simulink model "q1_model2"  (R2018a)
settings: Solver=FixedStepAuto  StartTime=0.0  StopTime=t_f  FixedStep=1  RelTol=1e-3
values from neighbouring files (symbols this model uses):
  A = [100  0  0  -57.735026919; 0  100  0  -57.735026919; 0  0  100  -57.735026919]    [data.mat]    (also in q1.m = [h1_hat h2_hat h3_hat h4_hat])
  I_b = [100 1 2; 1 150 3; 2 3 200]    [q1.m]    (also in q3.m)
  Kd = -4    [q1.m]
  Kp = -.01    (= -0.01)    [q1.m]
  omega_B_N_t0 = zeros(3,1)    [q1.m]
  pinvA = pinv(A)    [q1.m]
  q_f = [q_f(2:4) q_f(1)].'    [q1.m]
  q_t0 = [0 0 0 1].'    [q1.m]    (also in q3.m)
libraries: vrlib x1
settings Model: Creator=Padraig Lysandrou  LastModifiedBy=Padraig Lysandrou

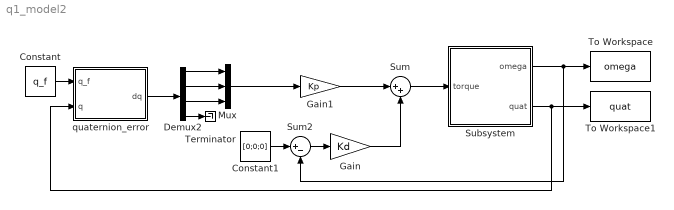
== system q1_model2 ==
  Constant : Constant  Value=q_f  VectorParams1D=off
  Constant1 : Constant  Value=[0;0;0]
  Demux2 : Demux
  Gain : Gain  Gain=Kd
  Gain1 : Gain  Gain=Kp
  Mux : Mux  Inputs=3
  Subsystem : Subsystem
  Sum : Sum  Inputs=|++
  Sum2 : Sum  Inputs=|+-
  Terminator : Terminator
  To Workspace : ToWorkspace  VariableName=omega  SaveFormat=Timeseries  SampleTime=-1
  To Workspace1 : ToWorkspace  VariableName=quat  SaveFormat=Timeseries  SampleTime=-1
  quaternion_error : MATLAB Function  TreatAsAtomicUnit=on
  wires:
  Sum/1 -> Subsystem/1(torque)
  Subsystem/1("omega ") -> Sum2/2, To Workspace/1
  Gain1/1 -> Sum/1
  Gain/1 -> Sum/2
  Constant1/1 -> Sum2/1
  Sum2/1 -> Gain/1
  Subsystem/2(quat) -> quaternion_error/2(q), To Workspace1/1
  Constant/1 -> quaternion_error/1(q_f)
  Demux2/3 -> Mux/3
  Demux2/1 -> Mux/1
  Demux2/4 -> Terminator/1
  Demux2/2 -> Mux/2
  quaternion_error/1(dq) -> Demux2/1
  Mux/1 -> Gain1/1

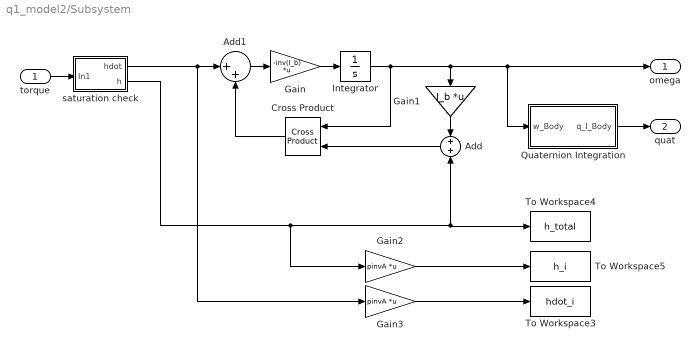
== system q1_model2/Subsystem ==
  torque : Inport
  Add : Sum
  Add1 : Sum  Inputs=|++
  Cross Product : vrlib/Utilities/Cross Product
      settings: SourceProductBaseCode=VR
  Gain : Gain  Gain=-inv(I_b)  Multiplication=Matrix(K*u) (u vector)
  Gain1 : Gain  Gain=I_b  Multiplication=Matrix(K*u) (u vector)
  Gain2 : Gain  Gain=pinvA  Multiplication=Matrix(K*u) (u vector)
  Gain3 : Gain  Gain=pinvA  Multiplication=Matrix(K*u) (u vector)
  Integrator : Integrator  InitialCondition=omega_B_N_t0
  Quaternion Integration : Subsystem
  To Workspace3 : ToWorkspace  VariableName=hdot_i  SaveFormat=Timeseries  SampleTime=-1
  To Workspace4 : ToWorkspace  VariableName=h_total  SaveFormat=Timeseries  SampleTime=-1
  To Workspace5 : ToWorkspace  VariableName=h_i  SaveFormat=Timeseries  SampleTime=-1
  saturation check : Subsystem
  "omega " : Outport
  quat : Outport  Port=2
  wires:
  Integrator/1 -> Quaternion Integration/1(w_Body), "omega "/1, Gain1/1, Cross Product/1
  Gain/1 -> Integrator/1
  Gain1/1 -> Add/1
  Add/1 -> Cross Product/2
  Add1/1 -> Gain/1
  Cross Product/1 -> Add1/2
  saturation check/2(h) -> Gain2/1, Add/2, To Workspace4/1
  Gain2/1 -> To Workspace5/1
  Gain3/1 -> To Workspace3/1
  Quaternion Integration/1(q_I_Body) -> quat/1
  torque/1 -> saturation check/1(In1)
  saturation check/1(hdot) -> Gain3/1, Add1/1

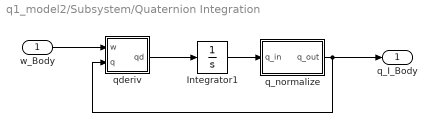
== system q1_model2/Subsystem/Quaternion Integration ==
  w_Body : Inport
  Integrator1 : Integrator  InitialCondition=q_t0
  q_normalize : Subsystem
  qderiv : Subsystem
  q_I_Body : Outport
  wires:
  w_Body/1 -> qderiv/1(w)
  q_normalize/1(q_out) -> qderiv/2(q), q_I_Body/1
  Integrator1/1 -> q_normalize/1(q_in)
  qderiv/1(qd) -> Integrator1/1

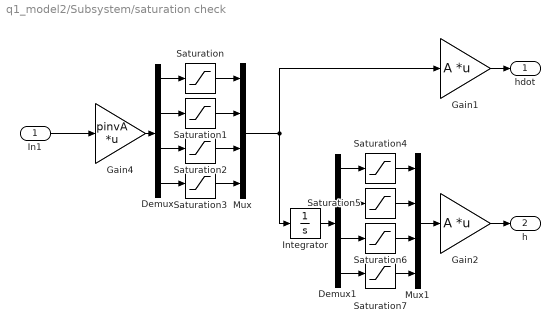
== system q1_model2/Subsystem/saturation check ==
  In1 : Inport
  Demux : Demux
  Demux1 : Demux
  Gain1 : Gain  Gain=A  Multiplication=Matrix(K*u) (u vector)
  Gain2 : Gain  Gain=A  Multiplication=Matrix(K*u) (u vector)
  Gain4 : Gain  Gain=pinvA  Multiplication=Matrix(K*u) (u vector)
  Integrator : Integrator
  Mux : Mux
  Mux1 : Mux
  Saturation{,1..3} (4 alike) : Saturate  UpperLimit=0.0002  LowerLimit=-0.0002
  Saturation{4..7} (4 alike) : Saturate  UpperLimit=0.0087  LowerLimit=-0.0087
  hdot : Outport
  h : Outport  Port=2
  wires:
  Demux/1 -> Saturation/1
  Demux/2 -> Saturation1/1
  Demux/3 -> Saturation2/1
  Demux/4 -> Saturation3/1
  Saturation/1 -> Mux/1
  Saturation1/1 -> Mux/2
  Saturation2/1 -> Mux/3
  Saturation3/1 -> Mux/4
  Mux/1 -> Gain1/1, Integrator/1
  Gain4/1 -> Demux/1
  In1/1 -> Gain4/1
  Gain1/1 -> hdot/1
  Integrator/1 -> Demux1/1
  Demux1/1 -> Saturation4/1
  Demux1/2 -> Saturation5/1
  Demux1/3 -> Saturation6/1
  Demux1/4 -> Saturation7/1
  Saturation4/1 -> Mux1/1
  Saturation5/1 -> Mux1/2
  Saturation6/1 -> Mux1/3
  Saturation7/1 -> Mux1/4
  Mux1/1 -> Gain2/1
  Gain2/1 -> h/1

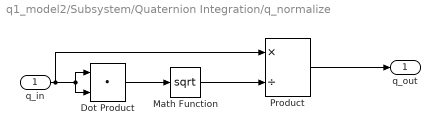
== system q1_model2/Subsystem/Quaternion Integration/q_normalize ==
  q_in : Inport  PortDimensions=4
  Dot Product : DotProduct  InputSameDT=on  OutDataTypeStr=Inherit: Inherit via internal rule
  Math Function : Math  Operator=sqrt  SaturateOnIntegerOverflow=on
  Product : Product  Inputs=*/  SaturateOnIntegerOverflow=on  InputSameDT=on  OutDataTypeStr=Inherit: Same as first input
  q_out : Outport
  wires:
  Product/1 -> q_out/1
  Math Function/1 -> Product/2
  Dot Product/1 -> Math Function/1
  q_in/1 -> Dot Product/2, Dot Product/1, Product/1

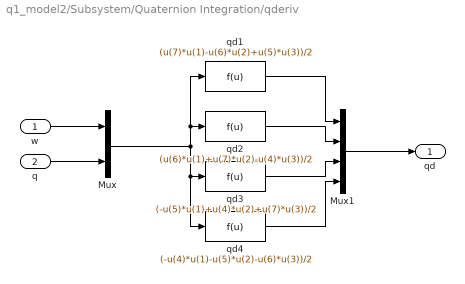
== system q1_model2/Subsystem/Quaternion Integration/qderiv ==
  w : Inport
  q : Inport  Port=2
  Mux : Mux  Inputs=2
  Mux1 : Mux
  qd1 : Fcn  Expr=(u(7)*u(1)-u(6)*u(2)+u(5)*u(3))/2
  qd2 : Fcn  Expr=(u(6)*u(1)+u(7)*u(2)-u(4)*u(3))/2
  qd3 : Fcn  Expr=(-u(5)*u(1)+u(4)*u(2)+u(7)*u(3))/2
  qd4 : Fcn  Expr=(-u(4)*u(1)-u(5)*u(2)-u(6)*u(3))/2
  qd : Outport
  wires:
  Mux1/1 -> qd/1
  qd4/1 -> Mux1/4
  qd3/1 -> Mux1/3
  qd2/1 -> Mux1/2
  qd1/1 -> Mux1/1
  Mux/1 -> qd4/1, qd3/1, qd2/1, qd1/1
  q/1 -> Mux/2
  w/1 -> Mux/1

== matlab function q1_model2/quaternion_error ==
  data: q_f input; q input; dq output
function dq = quaterr(q_f, q)
dq = zeros(4,1);
quatmult = zeros(4,1);
quatmult = [q(4)*eye(3) q(1:3); -q(1:3).' q(4)]*[-q_f(1:3); q_f(4)];
dq = -(1/(q_f(4)^2 + q_f(1)^2 + q_f(2)^2 + q_f(3)^2))*quatmult;
end
